simulink model "notch_filter"  (R2020a)
settings: Solver=FixedStepAuto  StartTime=0.0  StopTime=duration  FixedStep=deltaT  RelTol=1e-3
values from neighbouring files (symbols this model uses):
  A = 1    [dataAnalisys.m]
  Q = 1    [dataAnalisys.m]
  w = omega(i)    [dataAnalisys.m]
  w0 = 60    [dataAnalisys.m]
  wz = 60    [dataAnalisys.m]
settings Model: Creator=acer  LastModifiedBy=acer

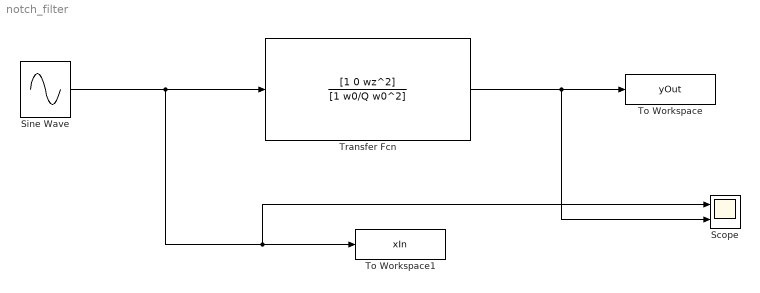
== system notch_filter ==
  Scope : Scope  NumInputPorts=2
  Sine Wave : Sin  Amplitude=A  Frequency=w  SampleTime=0
  To Workspace : ToWorkspace  VariableName=yOut  SampleTime=-1
      settings: Save2DSignal=2-D array (concatenate along first dimension)
  To Workspace1 : ToWorkspace  VariableName=xIn  SampleTime=-1
      settings: Save2DSignal=2-D array (concatenate along first dimension)
  Transfer Fcn : TransferFcn  Numerator=[1 0 wz^2]  Denominator=[1 w0/Q w0^2]
  wires:
  Sine Wave/1 -> Scope/1, To Workspace1/1, Transfer Fcn/1
  Transfer Fcn/1 -> Scope/2, To Workspace/1
